simulink model "lab"  (R2017a)
settings: Solver=VariableStepAuto  StartTime=0.0  StopTime=60  RelTol=1e-3
values from neighbouring files (symbols this model uses):
  K1 = 1    [lab_params.m]
  K2 = 10    [lab_params.m]
  K3 = 100    [lab_params.m]
settings Model: Creator=adityaaaap  LastModifiedBy=adityaaaap

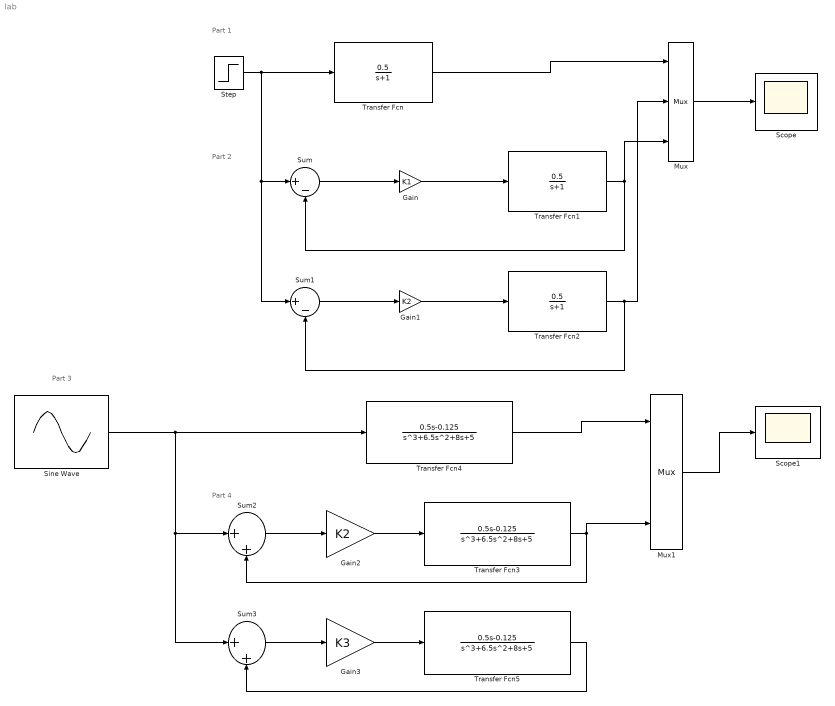
== system lab ==
  note: Part 3
  note: Part 1
  note: Part 2
  note: Part 4
  Gain : Gain  Gain=K1
  Gain1 : Gain  Gain=K2
  Gain2 : Gain  Gain=K2
  Gain3 : Gain  Gain=K3
  Mux : Mux  Inputs=3
  Mux1 : Mux  Inputs=3
  Scope : Scope
  Scope1 : Scope
  Sine Wave : Sin  Frequency=0.1  SampleTime=0
  Step : Step  Time=0  SampleTime=0
  Sum : Sum  Inputs=|+-
  Sum1 : Sum  Inputs=|+-
  Sum2 : Sum  Inputs=|++
  Sum3 : Sum  Inputs=|++
  Transfer Fcn : TransferFcn  Numerator=[0.5]  Denominator=[1 1]
  Transfer Fcn1 : TransferFcn  Numerator=[0.5]  Denominator=[1 1]
  Transfer Fcn2 : TransferFcn  Numerator=[0.5]  Denominator=[1 1]
  Transfer Fcn3 : TransferFcn  Numerator=[0.5 -0.125]  Denominator=[1 6.5 8 5]
  Transfer Fcn4 : TransferFcn  Numerator=[0.5 -0.125]  Denominator=[1 6.5 8 5]
  Transfer Fcn5 : TransferFcn  Numerator=[0.5 -0.125]  Denominator=[1 6.5 8 5]
  wires:
  Step/1 -> Sum1/1, Sum/1, Transfer Fcn/1
  Gain/1 -> Transfer Fcn1/1
  Sum/1 -> Gain/1
  Transfer Fcn/1 -> Mux/1
  Transfer Fcn1/1 -> Sum/2, Mux/3
  Mux/1 -> Scope/1
  Transfer Fcn2/1 -> Mux/2, Sum1/2
  Gain1/1 -> Transfer Fcn2/1
  Sum1/1 -> Gain1/1
  Sine Wave/1 -> Sum3/1, Sum2/1, Transfer Fcn4/1
  Transfer Fcn4/1 -> Mux1/1
  Mux1/1 -> Scope1/1
  Sum2/1 -> Gain2/1
  Gain2/1 -> Transfer Fcn3/1
  Transfer Fcn3/1 -> Sum2/2, Mux1/3
  Sum3/1 -> Gain3/1
  Transfer Fcn5/1 -> Sum3/2
  Gain3/1 -> Transfer Fcn5/1
